simulink model "simulink_s1"  (R2024a)
settings: Solver=VariableStepAuto  StartTime=0.0  StopTime=11.25  RelTol=1e-3
undefined symbols (not defined in the file): OUT, REF
settings Model: Creator=Admin  LastModifiedBy=ajj
settings SolverCC: AlgebraicLoopSolver=TrustRegion
settings RTWCC: GPUComputeCapability=3.5

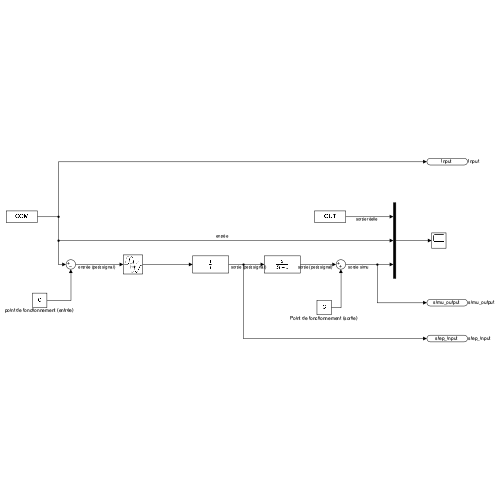
[thumbnail: Simulink's stored preview of the top-level diagram]
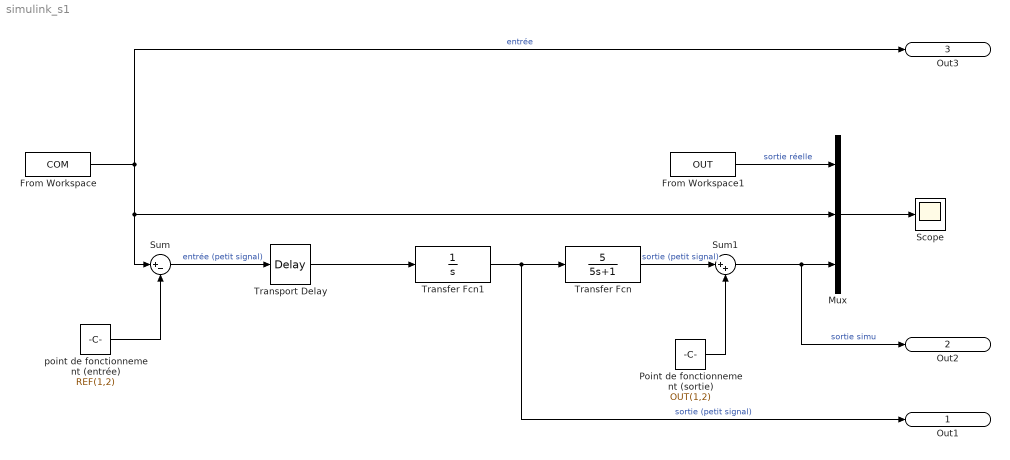
== system simulink_s1 ==
  From Workspace : FromWorkspace  VariableName=COM
  From Workspace1 : FromWorkspace  VariableName=OUT
  Mux : Mux  Inputs=3
  Point de fonctionnement (sortie) : Constant  Value=OUT(1,2)
  Scope : Scope
  Sum : Sum  Inputs=|+-
  Sum1 : Sum  Inputs=|++
  Transfer Fcn : TransferFcn  Numerator=[5]  Denominator=[ 5 1 ]
  Transfer Fcn1 : TransferFcn  Denominator="[ 1  0]"
  Transport Delay : TransportDelay  DelayTime=2
  point de fonctionnement (entrée) : Constant  Value=REF(1,2)
  Out1 : Outport  SignalName=step_input
  Out2 : Outport  Port=2  SignalName=simu_output
  Out3 : Outport  Port=3  SignalName=Input
  wires:
  Sum/1 -> Transport Delay/1  "entrée (petit signal)"
  From Workspace1/1 -> Mux/1  "sortie réelle"
  From Workspace/1 -> Sum/1, Mux/2, Out3/1  "entrée"
  Transfer Fcn/1 -> Sum1/1  "sortie (petit signal)"
  Mux/1 -> Scope/1
  Point de fonctionnement (sortie)/1 -> Sum1/2
  point de fonctionnement (entrée)/1 -> Sum/2
  Sum1/1 -> Out2/1, Mux/3  "sortie simu"
  Transfer Fcn1/1 -> Out1/1, Transfer Fcn/1  "sortie (petit signal)"
  Transport Delay/1 -> Transfer Fcn1/1
